simulink model "larix2_tuner_closedLoop"  (R2020b)
settings: Solver=FixedStepDiscrete  StartTime=0.0  StopTime=20  FixedStep=0.002  RelTol=1e-3
PostLoadFcn:
  | load('ThrustTable.mat');
  | init();
values from neighbouring files (symbols this model uses):
  blimp = inertias()    [init.m]
  eul_0 = [-45*pi/180 0 0]    [init.m]
  FLRS3_0 = [0 0 0 0]    [init.m]
  g = 9.810    (= 9.81)    [init.m]
  omega_0 = [0 0 0]    [init.m]
  pos_0 = [0 0 0]    [init.m]
  vel_0 = [0 0 0]    [init.m]
undefined symbols (not defined in the file or in its folder): DiscIntNeverNeededParam
libraries: slpidlib x10, simulink x10, sharedtransform x3, vrlib x3
(part 2 of 2)

== matlab function larix2_tuner_closedLoop/Dynamics Model/Dynamics (NED) ==
  data: F input; x_dotdot output; e input; x_dot input
function x_dotdot = fcn(F,e,x_dot)

fL = F(1);
fR = F(2);
stick = -F(3);
fB = F(4);

roll = e(1);
pitch = e(2);
yaw = e(3);
%e3 = e(4);


u = x_dot(1);
v = x_dot(2);
w = x_dot(3);
p = x_dot(4);
q = x_dot(5);
r = x_dot(6);

%}

g = 9.81;
rho_air = 1.225; 
eta_air = 1.802e-5;



blimp = inertias();
prp = blimp.prp;
par = blimp.par;
in = blimp.mM;




mx = in.M(1,1);
my = in.M(2,2);
mz = in.M(3,3);

Jxx = in.M(4,4);
Jyy = in.M(5,5);
Jzz = in.M(6,6);
Jxz = in.M(3,6);
 
%DYNAMICS

%{
f1 = -mz*w*q + my*r*v + in.mass*(in.CG(1)*( q^2 + r^2) - in.CG(3)*r*p);
f2 = -mx*u*r + mz*p*w + in.mass*(-in.CG(1)*p*q - in.CG(3)*r*q);
f3 = -my*v*p + mx*q*u + in.mass*(-in.CG(1)*r*p + in.CG(3)*(q^2 + p^2));
f4 = -(Jzz - Jyy)*r*q + Jxz*p*q + in.mass*in.CG(3)*(u*r - p*w);
f5 = -(Jxx - Jzz)*p*r + Jxz*(r^2 - p^2) + in.mass*(in.CG(1)*(v*p - q*u) - in.CG(3)*(w*q - r*v));
f6 = -(Jyy - Jxx)*q*p - Jxz*q*r + in.mass*(-in.CG(1)*(u*r - p*w));
F = [f1; f2; f3; f4; f5; f6];
%}
%%{
F = -[in.mass*(cross([p q r]',diag(in.M(1:3,1:3)).*[u v w]')+cross([p q r]',cross([p q r]',in.CG)')); ...
    cross([p q r]',(in.inertia*[p q r]'))+cross(in.mass*in.CG',cross([p q r]',[u v w]'))];
%}
%GRAVITATIONAL FORCES Quaternion
%{
DCM = [e0^2+e1^2-e2^2-e3^2, 2*(e1*e2-e0*e3),2*(e0*e2-e1*e3);...
        2*(e0*e3-e1*e2),e0^2-e1^2+e2^2-e3^2,2*(e2*e3-e0*e1);...
        2*(e1*e3-e0*e2),2*(e0*e1-e2*e3),e0^2-e1^2-e2^2+e3^2];


    
G = [DCM(3,1)*(W+B); DCM(3,2)*(W+B); DCM(3,3)*(W+B);DCM(3,2)*in.a(3)*W; (DCM(3,1)*in.a(3)-DCM(3,3)*in.a(1))*W; DCM(3,2)*in.a(1)*W];
%}



%GRAVITATIONAL FORCES EULER
%{
g_vec = [0 0 g]';

%rot = eul2rotm([e0 e1 e2],'XYZ')';
rot = eul2rotm([roll pitch yaw],'XYZ')';

G_forces = [0 0 h]'*rot*g_vec;

gondola_mass = par.gondola_body.mass + par.gondola_support.mass + par.stick.mass + 2*par.blade_left.mass;      %mass of the whole gondola assembly with its CG at [CG_stick_x 0 CG_stick_z]

G_gondola = gondola_mass*rot*g_vec;


CG_ga = par.stick.position';    %CG coordinates from CV to Gondola assembly

G_moments = cross(G_gondola, CG_ga);

G = [G_forces; G_moments];
%}

h = prp.mass_H;
B = prp.volume_blimp_body*prp.density_air*g;
W = B + h*g;
%%{
rot = eul2rotm([roll pitch yaw],'XYZ');
b_offset = 0;

G = [rot(3,1)*(W-B), rot(3,2)*(W-B), rot(3,3)*(W-B), -rot(3,2)*(in.CG(3)+b_offset)*W, (rot(3,1)*(in.CG(3)+b_offset) - rot(3,3)*in.CG(1))*W, rot(3,2)*in.CG(1)*W]';
%}
%{
g_vec = [0 0 g];

rotNEDtoBF = eul2rotm([roll pitch yaw],'XYZ')';

g_bf = g_vec*rotNEDtoBF;

G = [h*g_bf, cross(in.CG,W*g_bf)]';
%}


%PROPULSION FORCES


rL = blimp.par.blade_left.position';
rR = blimp.par.blade_right.position';
rB = blimp.par.bot_rud_motor.position';

FL = fL*[sin(-stick*pi/2) 0 cos(-stick*pi/2)]';
FR = fR*[sin(-stick*pi/2) 0 cos(-stick*pi/2)]';
FB = fB*[0 1 0]';

TL = cross(rL,FL);
TR = cross(rR,FR);
TB = cross(rB,FB);
 
Forces = FL+FR+FB;
Torques = TL+TR+TB;

P_NED = [Forces;Torques];

%P = P_NED.*[1 1 -1 1 1 -1]';        %convert P from NEU (allocation) to NED 
P = P_NED;

% AERO FORCES

%AR ~= 0.7 --> nu_fin (Modeling and Simulation of Airship Dynamics)
%finenessratio = 2.375
%hull projected area = 7.461m^2   effective fin area = 0.64 m^2
% effective fin area/ hull projected area = 0.086 --> nu hull

nu_hull =  1.01;
nu_fin = 0.58;

L_f = (blimp.prp.length_rud_part1+blimp.prp.length_rud_part2);
D_f = blimp.prp.height_rud_part1;
L_h = prp.length_blimp_body;
D_h = 2*prp.radius_blimp_body;

Re_0h = abs(u)*prp.length_blimp_body*rho_air/eta_air;
Re_0f = abs(u)*L_f*rho_air/eta_air;

if u == 0
    Cf = 0;
    Cdf0 = 0;
else
Cf = 0.045*Re_0h^(-1/6);
Cdf0 = 1.328/sqrt(Re_0f)+8.25/Re_0f;
end

Cdh0 = Cf*(4*(L_h/D_h)^(1/3)+6*(D_h/L_h)^(-1.2)+24*(D_h/L_h)^(-2.7));
Cdhc = 0.6845;
Cdfc = (1.1+(L_f/D_f+D_f/L_f)*0.02);
Cdg0 = 1.05;
Cdgc = 1.05;


e = sqrt((prp.length_blimp_a1^2 + prp.radius_blimp_body^2)/prp.length_blimp_a1);

S = pi*prp.radius_blimp_body*(prp.radius_blimp_body+(prp.length_blimp_a1^2)*sin(e)/e);

Vh_ref = prp.volume_blimp_body; %volume based on two semi ellipsoids
Sg_ref = prp.volume_gondola_body^(2/3);
Sh_ref = Vh_ref^(2/3);
%Sf_ref = 2*prp.surface_two_fins;
Sf_ref = (2*prp.width_rud_part1*(prp.length_rud_part1*prp.height_rud_part1+prp.length_rud_part2*prp.height_rud_part2))^(2/3);


fh = (prp.length_tip_to_fin - prp.length_blimp_a1)/prp.length_blimp_a2;
xcv = prp.length_blimp_a1+(3/8)*(prp.length_blimp_a2-prp.length_blimp_a1);
Xcv2=-(3/8)*(prp.length_blimp_a2-prp.length_blimp_a1);
xcv=Xcv2;
%xcv = prp.length_blimp_a1 - (4*pi/3)*(prp.length_blimp_a1-prp.length_blimp_a2);

I_1 = pi*((prp.radius_blimp_body^2)/Sh_ref)*(1-fh^2);
I_3 = pi*((prp.radius_blimp_body^2)/(3*prp.length_blimp_body*Sh_ref)*(prp.length_blimp_a1 - 2*prp.length_blimp_a2*(fh^3) - 3*prp.length_blimp_a1*(fh^2)) - xcv*I_1/prp.length_blimp_body);


J_1 = prp.radius_blimp_body/(2*Sh_ref)*(pi*prp.length_blimp_a1 + prp.length_blimp_a2*sqrt(1-fh^2)*fh + 2*prp.length_blimp_a2*asin(fh));
J_2 = (J_1/prp.length_blimp_body)*(prp.length_blimp_a1-xcv) + (2*prp.radius_blimp_body/(3*prp.length_blimp_body*Sh_ref))*(prp.length_blimp_a2^2 - prp.length_blimp_a1^2 - (prp.length_blimp_a2^2)*(1-fh^2)^(3/2));

%reference length normalization
%{
L = L_h;
D=D_h;
lf1 = prp.length_tip_to_ac_fin/L;            %tip to aero center of fin
lf2 = prp.length_tip_to_gc_fin/L;              %tip to geo center of fin
lf3 = prp.length_yz_origin_to_ac_fin/L;
lgx= par.gondola_body.position(1)/L;
lgz= par.gondola_body.position(3)/L;

Sf_ref= Sf_ref/Sh_ref;
Sg_ref= Sg_ref/Sh_ref;
%}



L = L_h;
D=D_h;
lf1 = prp.length_tip_to_ac_fin;            %tip to aero center of fin
lf2 = prp.length_tip_to_gc_fin;              %tip to geo center of fin
lf3 = prp.length_yz_origin_to_ac_fin;
lgx= par.gondola_body.position(1);
lgz= par.gondola_body.position(3);
Sf_ref= Sf_ref;
Sg_ref= Sg_ref;

U_abs = sqrt(u^2 +v^2 +w^2);

a = atan2(w,u);


LS = liftslope(abs(a));


if U_abs == 0
    b = 0;
else
    b = asin(v/U_abs);
end

%revised model

%{
Cx1 = -(Cdh0* + Cdf0*Sf_ref + Cdg0*Sg_ref);
Cx2 = (in.k(2)-in.k(1))*nu_hull*I_1*Sh_ref;          %VLT l1 ???
Cx3 = 0;

Cy1 = -Cx2;                                       
Cy2 = -0.5*LS*Sf_ref*nu_fin;                               %dCl/da = 2*pi  --> only for small angle of attack     from On the lift curve slope for rectangular flat plate wings at moderate Reynolds number
Cy3 = -(Cdhc*J_1+Cdfc*Sf_ref + Cdgc*Sg_ref);
Cy4 = 0;

Cz1 = -Cx2;
Cz2 = Cy2;
Cz3 = -(Cdhc*J_1 + Cdfc*Sf_ref);       
Cz4 = Cy4;

Cl1 = 0;
Cl2 = -Cdgc*Sg_ref*lgz;
Cl3 = Cl2;
Cl4 = -(Cdgc*Sg_ref*lgz + Cdfc*Sf_ref*lf3);

Cm1 = -(in.k(2)-in.k(1))*nu_hull*I_3;
Cm2 = -0.5*LS*Sf_ref*nu_fin*lf1;
Cm3 = -(Cdhc*J_2+ Cdfc*Sf_ref*lf2);
Cm4 = 0;
Cm5 = -Cdfc*Sf_ref*lf2;


Cn1 = -Cm1;
Cn2 = -Cm2;
Cn3 = (Cdhc*J_2 + Cdfc*Sf_ref*lf2 + Cdgc*Sg_ref*lgx);
Cn4 = -Cm4;
Cn5 = -(Cdfc*Sf_ref*lf2 + Cdgc*Sg_ref*lgx);

X = 0.5*rho_air*(U_abs^2)*Sh_ref*(Cx1*(-sign(u))*(cos(a)^2)*(cos(b)^2) + Cx2*sin(2*a)*sin(a/2)+Cx3);
Y = 0.5*rho_air*(U_abs^2)*Sh_ref*(Cy1*cos(b/2)*sin(2*b)+Cy2*sin(2*b) + Cy3*sin(b)*sin(abs(b)));
Z = 0.5*rho_air*(U_abs^2)*Sh_ref*(Cz1*cos(a/2)*sin(2*a)+Cz2*sin(2*a) + Cz3*sin(a)*sin(abs(a)));

L = 0.5*rho_air*(U_abs^2)*L*Sh_ref*(Cl1 + Cl2*(sin(b)*sin(abs(b)))) + 0.5*rho_air*Sh_ref*L*(((L^3)*Cl3*r*abs(r) + (D^2)*Cl4*p*abs(p)));
M = 0.5*rho_air*(U_abs^2)*L*Sh_ref*(Cm1*cos(a/2)*sin(2*a) + Cm2*sin(2*a) + Cm3*sin(a)*sin(abs(a)) + Cm4) + 0.5*rho_air*Sh_ref*(L^3)*Cm5*q*abs(q) -Xcv2*Z ;
N = 0.5*rho_air*(U_abs^2)*L*Sh_ref*(Cn1*cos(b/2)*sin(2*b) + Cn2*sin(2*b) + Cn3*sin(b)*sin(abs(b)) + Cn4) + 0.5*rho_air*Sh_ref*(L^3)*Cn5*r*abs(r) +Xcv2*Y;
%}

%%{

Cx1 = -(Cdh0*Sh_ref + Cdf0*Sf_ref + Cdg0*Sg_ref);
Cx2 = (in.k(2)-in.k(1))*nu_hull*I_1*Sh_ref;             %munk lift
Cx3 = 0;

Cy1 = -Cx2;                                       
Cy2 = -0.5*LS*Sf_ref*nu_fin;                               %dCl/da = 2*pi  --> only for small angle of attack     from On the lift curve slope for rectangular flat plate wings at moderate Reynolds number
Cy3 = -(Cdhc*J_1*Sh_ref+Cdfc*Sf_ref + Cdgc*Sg_ref);
Cy4 = 0;

Cz1 = -Cx2;
Cz2 = Cy2;
Cz3 = -(Cdhc*J_1*Sh_ref + Cdfc*Sf_ref);       
Cz4 = Cy4;

Cl1 = 0;
Cl2 = Cdgc*Sg_ref*lgz;
Cl3 = Cdgc*Sg_ref*lgz*prp.length_blimp_body^2;
Cl4 = -(Cdgc*Sg_ref*lgz + Cdfc*Sf_ref*lf3)*(2*prp.radius_blimp_body)^2;

Cm1 = -(in.k(2)-in.k(1))*nu_hull*I_3*Sh_ref*prp.length_blimp_body;
Cm2 = -0.5*LS*Sf_ref*nu_fin*lf1;
Cm3 = -(Cdhc*J_2*Sh_ref*prp.length_blimp_body + Cdfc*Sf_ref*lf2);
Cm4 = 0;
Cm5 = -Cdfc*Sf_ref*lf2*(prp.length_blimp_body^2);


Cn1 = -Cm1;
Cn2 = -Cm2;
Cn3 = (Cdhc*J_2*Sh_ref*prp.length_blimp_body + Cdfc*Sf_ref*lf2 + Cdgc*Sg_ref*lgx);
Cn4 = -Cm4;
Cn5 = -(Cdfc*Sf_ref*lf2 + Cdgc*Sg_ref*lgx)*(prp.length_blimp_body^2);

%Cm5 = 0;
%Cn5 = 0;  
    
%e = sqrt(((prp.length_blimp_body*0.5)*(prp.length_blimp_body*0.5)-prp.radius_blimp_body*prp.radius_blimp_body)/(prp.length_blimp_body*0.5));



%{

X = 0.5*rho_air*(U_abs^2)*(Cx1*(cos(a)^2)*(cos(b)^2) + Cx2*sin(2*a)*sin(a/2));
Y = 0.5*rho_air*(U_abs^2)*(Cy1*cos(b/2)*sin(2*b)+Cy2*sin(2*b) + Cy3*sin(b)*sin(abs(b)));
Z = 0.5*rho_air*(U_abs^2)*(Cz1*cos(a/2)*sin(2*a)+Cz2*sin(2*a) + Cz3*sin(a)*sin(abs(a)));

L = 0.5*rho_air*(U_abs^2)*(0.5*rho_air*S*Cl3*p*abs(p));
M = 0.5*rho_air*(U_abs^2)*(Cm1*cos(a/2)*sin(2*a)+Cm2*sin(2*a)+Cm3*sin(a)*sin(abs(a))+0.5*rho_air*S*Cm5*q*abs(q));
N = 0.5*rho_air*(U_abs^2)*(Cn1*cos(b/2)*sin(2*b)+Cn2*sin(2*b)+Cn3*sin(b)*sin(abs(b))+0.5*rho_air*S*Cn5*r*abs(r));

%}

X = 0.5*rho_air*(U_abs^2)*S*(Cx1*sign(u)*(cos(a)^2)*(cos(b)^2) + Cx2*(sin(2*a)*sin(a/2)+sin(2*b)*sin(b/2)+Cx3));
Y = 0.5*rho_air*(U_abs^2)*S*(Cy1*cos(b/2)*sin(2*b)+Cy2*sin(2*b) + Cy3*sin(b)*sin(abs(b)));
Z = 0.5*rho_air*(U_abs^2)*S*(Cz1*cos(a/2)*sin(2*a)+Cz2*sin(2*a) + Cz3*sin(a)*sin(abs(a)));

L = 0.5*rho_air*(U_abs^2)*prp.length_blimp_body*S*(Cl1 + Cl2*(sin(b)*sin(abs(b))) + 0.5*rho_air*S*(Cl3*r*abs(r) + Cl4*p*abs(p)));
M = 0.5*rho_air*(U_abs^2)*prp.length_blimp_body*S*(Cm1*cos(a/2)*sin(2*a) + Cm2*sin(2*a) + Cm3*sin(a)*sin(abs(a)) + Cm4 + 0.5*rho_air*S*Cm5*q*abs(q));
N = 0.5*rho_air*(U_abs^2)*prp.length_blimp_body*S*(Cn1*cos(b/2)*sin(2*b) + Cn2*sin(2*b) + Cn3*sin(b)*sin(abs(b)) + Cn4 + 0.5*rho_air*S*Cn5*r*abs(r));

%Y = 0;
%L = 0;
%N = 0;

%}
 
A = [X;Y;Z;L;M;N];

%masstest = eye(6);
F_sum = (G+F+A+P);

%F_sum(3) = 0;
%F_sum(5) = 0;


%x_dotdot = in.M\(F_sum);
x_dotdot = in.M_inv*(F_sum);
end

== matlab function larix2_tuner_closedLoop/Actuator Allocation/acc_allocation ==
  data: euler input; acc_cmd input; F output size=4; blimp parameter
function F = fcn(euler, acc_cmd, blimp)

% accellerations in BFG cs
u_dot = acc_cmd(1);
%v_dot = acc_cmd(2);
w_dot = acc_cmd(3);
p_dot = acc_cmd(4);  
%q_dot = acc_cmd(5);
r_dot = acc_cmd(6);

roll = euler(1);
pitch = euler(2);


%ALLOCATION
                            % [-1 1]        stick accounts for pitch movement -> stays level
if w_dot <= 0
    Thrustvector_angle = atan2(-(w_dot/cos(roll)),u_dot)*2/pi -1;  %neg towards front
else
    Thrustvector_angle = atan2(-(w_dot/cos(roll)),u_dot)*2/pi +1;
end

stick = Thrustvector_angle - pitch*2/pi;

%TF_BFtoBFG = eul2rotm([roll pitch 0],'XYZ')';   

%normalized accelerations
u_dot_norm = u_dot;
w_dot_norm = w_dot/cos(roll);

p_dot_norm = p_dot/(cos(Thrustvector_angle)*blimp.prp.length_stick);
r_dot_norm = r_dot/(cos(roll)*(abs(blimp.par.bot_rud_motor.position(1))));

acc_norm = single([u_dot_norm, 0, w_dot_norm, p_dot_norm, 0, r_dot_norm]);
acc_norm(isnan(acc_norm)) = 0;

%inertia_ax_bfg = TF_BFtoBFG * blimp.mM.M(1:3,1:3) * TF_BFtoBFG';        %transform axial and rotational inertia into BFG coordinates
%inertia_rot_bfg = TF_BFtoBFG * blimp.mM.M(4:6,4:6) * TF_BFtoBFG';
inertia_ax_bfg = blimp.mM.M(1:3,1:3);        %transform axial and rotational inertia into BFG coordinates
inertia_rot_bfg = blimp.mM.M(4:6,4:6);


%multiply by mass matrix to get actual needed force
FT_norm = acc_norm.*[diag(inertia_ax_bfg); diag(inertia_rot_bfg)]';

FLRuw = sign(FT_norm(3))*sqrt(FT_norm(1)^2 + FT_norm(3)^2);
FLRp = FT_norm(4);
F3r = FT_norm(6);

F3 = F3r;
%F3= -0.18;
%F3= 0.7

%enforce saturation safety bounds


%if F3 comes too close to saturation, decrease delta FLR
%works for "u minmal v movement" and "u allowed v movement"
if (F3 < blimp.prp.FB_min*blimp.prp.FB_softboundmargin) && (blimp.prp.FB_min < F3) &&(FLRp > 0)
    delta_bound = (blimp.prp.FB_min - F3)/((1-blimp.prp.FB_softboundmargin)*blimp.prp.FB_min); % = distance from hard bound / distance from hard bound at the beginning of th safetymargin 
elseif (F3 > blimp.prp.FB_max*blimp.prp.FB_softboundmargin) && (blimp.prp.FB_max > F3)&& (FLRp < 0)
    delta_bound = (blimp.prp.FB_max - F3)/((1-blimp.prp.FB_softboundmargin)*blimp.prp.FB_max);
elseif (blimp.prp.FB_min > F3) && (FLRp > 0)
    F3 = blimp.prp.FB_min;
    delta_bound = single(0);
elseif (blimp.prp.FB_max < F3) && (FLRp < 0)
    F3 = blimp.prp.FB_max;
    delta_bound = single(0);
else
    delta_bound = single(1);
end
    FLRp = FLRp*(1-0.6*(1-delta_bound)^2);
    
    

if (FLRuw/2 + abs(FLRp/2)) > blimp.prp.FL_max*blimp.prp.FLR_safetymargin          %include case if maximum is passed?
    if FLRp > 0
        FRp = blimp.prp.FR_max*blimp.prp.FLR_safetymargin;          % set trust to the minimal possible value on the side where the blimp should move to
        FLp = -FLRp + blimp.prp.FR_max*blimp.prp.FLR_safetymargin;       %calculate trust on the left side so that the resulting torque still comes out to the desired value even tho the thrust on the other side has hit the bound
        if (FLp + FRp) < FLRuw                                              %make sure the offset between FL and FR is never greater than the desired up/forward force since that would mean drift
            FLp = FLRuw - blimp.prp.FR_max*blimp.prp.FLR_safetymargin;
        end
        if FLp < blimp.prp.FL_min*blimp.prp.FLR_safetymargin            
            FLp = blimp.prp.FL_min*blimp.prp.FLR_safetymargin;          %hard limit  --> doesnt mean control is lost
        end
    else       
        FLp = blimp.prp.FR_max*blimp.prp.FLR_safetymargin; 
        FRp = FLRp + blimp.prp.FL_max*blimp.prp.FLR_safetymargin;      % the same thing as before but for the other movement direction
        if (FLp + FRp) < FLRuw                                             
            FRp = FLRuw - blimp.prp.FR_max*blimp.prp.FLR_safetymargin;
        end
        if FRp < blimp.prp.FR_min*blimp.prp.FLR_safetymargin
            FRp = blimp.prp.FR_min*blimp.prp.FLR_safetymargin;
        end
    end
    FLRuw = FLRuw - (FLp + FRp);                                        %subtract the difference of left and right thrust from the uw thrust to ensure correct trust (no w drift)
else
    FLp = -FLRp/2;
    FRp = FLRp/2;
end

FL = FLRuw/2 + FLp; 
FR = FLRuw/2 + FRp; 


LRS3 = [FL FR stick F3];

F = LRS3(1,:)'
